simulink model "DAC"  (R2023a)
settings: Solver=FixedStepDiscrete  StartTime=0.0  StopTime=1  FixedStep=0.001  RelTol=1e-3
values from neighbouring files (symbols this model uses):
  D_C = 14    [constant.m]
  U_max = 5    [constant.m]
settings Model: Creator=Ilya_Andriyanov  LastModifiedBy=ПК

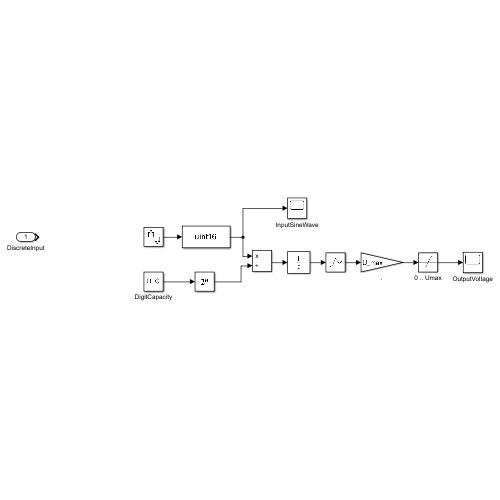
[thumbnail: Simulink's stored preview of the top-level diagram]
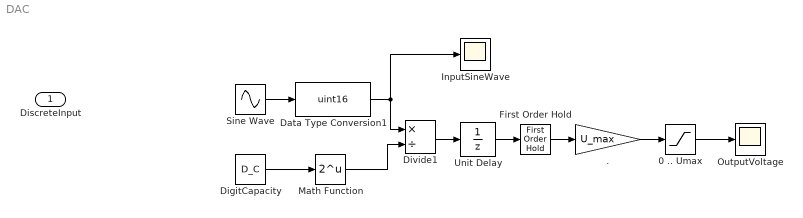
== system DAC ==
  DiscreteInput : Inport
  . : Gain  Gain=U_max
  0 .. Umax : Saturate  UpperLimit=U_max  LowerLimit=0
  Data Type Conversion1 : DataTypeConversion  OutDataTypeStr=uint16  SaturateOnIntegerOverflow=off  RndMeth=Floor
  DigitCapacity : Constant  Value=D_C
  Divide1 : Product  Inputs=*/
  First Order Hold : FirstOrderHold  ErrorTolerance=inf
  InputSineWave : Scope
  Math Function : Math  Operator=2^u
  OutputVoltage : Scope
  Sine Wave : Sin  Amplitude=2^D_C/2  Bias=2^D_C/2  Frequency=5  Phase=-pi/2  SampleTime=0.01
  Unit Delay : UnitDelay  SampleTime=-1  HasFrameUpgradeWarning=on
  wires:
  Math Function/1 -> Divide1/2
  0 .. Umax/1 -> OutputVoltage/1
  Divide1/1 -> Unit Delay/1
  DigitCapacity/1 -> Math Function/1
  ./1 -> 0 .. Umax/1
  Sine Wave/1 -> Data Type Conversion1/1
  Data Type Conversion1/1 -> InputSineWave/1, Divide1/1
  First Order Hold/1 -> ./1
  Unit Delay/1 -> First Order Hold/1
